simulink model "Sample594"  (R2021b)
settings: Solver=VariableStepAuto  StartTime=0.0  StopTime=10.0  RelTol=1e-3
undefined symbols (not defined in the file): DiscIntNeverNeededParam, magnitude, Newton, Raphson
libraries: simulink x402, pid_lib x98
(part 7 of 14)

== system Sample594/cfblk11/cfblk14/cfblk10/cfblk18 ==
  cfblk1 : Inport
  cfblk11 : Inport  Port=2
  cfblk12 : Inport  Port=3
  Action Port : ActionPort  ActionPortLabel=if(u1 >= 0)
  cfblk10 : Sin  TimeSource=Use external signal  SampleTime=0
  cfblk13 : Delay
  cfblk3 : DiscreteStateSpace  SampleTime=-1
  cfblk4 : pid_lib/PID Controller (2DOF)  Controller=PID  Form=Parallel  TimeDomain=Discrete-time  UseExternalTs=off  SampleTime=-1  IntegratorMethod=Forward Euler  FilterMethod=Forward Euler  ControllerParametersSource=internal  P=1  I=1  D=0  UseFilter=on  N=100  b=1  c=1  TunerSelectOption=Transfer Function Based (PID Tuner App)  InitialConditionSource=internal  InitialConditionForIntegrator=0  InitialConditionForFilter=0  DifferentiatorICPrevScaledInput=0  ExternalReset=none  TrackingMode=off  Kt=1  LimitOutput=off  SatLimitsSource=internal  UpperSaturationLimit=inf  LowerSaturationLimit=-inf  LinearizeAsGain=off  AntiWindupMode=none  Kb=1  POutMin=[]  POutMax=[]  IOutMin=[]  IOutMax=[]  DOutMin=[]  DOutMax=[]  NOutMin=[]  NOutMax=[]  bOutMin=[]  bOutMax=[]  cOutMin=[]  cOutMax=[]  SumOutMin=[]  SumOutMax=[]  SaturationOutMin=[]  SaturationOutMax=[]  PParamMin=[]  PParamMax=[]  IParamMin=[]  IParamMax=[]  DParamMin=[]  DParamMax=[]  NParamMin=[]  NParamMax=[]  bParamMin=[]  bParamMax=[]  cParamMin=[]  cParamMax=[]  KbParamMin=[]  KbParamMax=[]  KtParamMin=[]  KtParamMax=[]  KbOutMin=[]  KbOutMax=[]  KtOutMin=[]  KtOutMax=[]  IntegratorOutMin=[]  IntegratorOutMax=[]  FilterOutMin=[]  FilterOutMax=[]  SumI1OutMin=[]  SumI1OutMax=[]  SumI2OutMin=[]  SumI2OutMax=[]  SumI3OutMin=[]  SumI3OutMax=[]  SumI4OutMin=[]  SumI4OutMax=[]  SumDOutMin=[]  SumDOutMax=[]  Sum1OutMin=[]  Sum1OutMax=[]  Sum2OutMin=[]  Sum2OutMax=[]  Sum3OutMin=[]  Sum3OutMax=[]  DifferentiatorOutMin=[]  DifferentiatorOutMax=[]  FilterDiffOutCoefMin=[]  FilterDiffOutCoefMax=[]  ReciprocalOutMin=[]  ReciprocalOutMax=[]  SumDenOutMin=[]  SumDenOutMax=[]  SumNumOutMin=[]  SumNumOutMax=[]  DivideOutMin=[]  DivideOutMax=[]  UdiffTsProdOutMin=[]  UdiffTsProdOutMax=[]  NTsProdOutMin=[]  NTsProdOutMax=[]  UintegralTsProdOutMin=[]  UintegralTsProdOutMax=[]  UngainTsProdOutMin=[]  UngainTsProdOutMax=[]  IntegratorContinuousStateAttributes=''  IntegratorStateMustResolveToSignalObject=off  IntegratorRTWStateStorageClass=Auto  FilterContinuousStateAttributes=''  FilterStateMustResolveToSignalObject=off  FilterRTWStateStorageClass=Auto  ParallelPVariant=InternalParameters  IdealPVariant=Disabled  IVariant=InternalParameters  DVariant=InternalParameters  bVariant=InternalParameters  cVariant=InternalParameters  IntegratorVariant=Discrete  SatVariant=Disabled  AWVariant=Passthrough  PCopyVariant=Disabled  TRVariant=Disabled  FdbkBlocksVariant=Forward  IdealPFdbkVariant=Disabled  SatFdbkVariant=Disabled  DerivativeFilterVariant=ForwardEulerFilter  NVariant=InternalParameters  NCopyVariant=Disabled  FilterICVariant=InternalICsFilter  IntegratorICVariant=InternalICs  ExternalResetVariant=Disabled  TRSumVariant=Passthrough  SumFdbkVariant=Disabled  SumVariant=Sum_PID  TsampFilterVariant=InternalTs  TsampNgainVariant=Passthrough  TsampIntegralVariant=Passthrough  ExternalSaturationOutDataTypeStr=Inherit: Same as second input
      settings: SourceProductBaseCode=SL
  cfblk5 : simulink/Discrete/Transfer Fcn First Order  PoleZ=0.95  ICPrevOutput=0.0  DoSatur=off
  cfblk6 : Math  Operator=pow  SaturateOnIntegerOverflow=on
  cfblk7 : Gain  Gain=[178402085.468543]
  cfblk8 : Product
  cfblk9 : Trigonometry
  cfblk2 : Outport
  wires:
  cfblk1/1 -> cfblk10/1
  cfblk10/1 -> cfblk3/1, cfblk8/2
  cfblk3/1 -> cfblk2/1
  cfblk11/1 -> cfblk7/1
  cfblk9/1 -> cfblk4/1
  cfblk8/1 -> cfblk9/1
  cfblk12/1 -> cfblk6/1
  cfblk6/1 -> cfblk5/1
  cfblk7/1 -> cfblk6/2
  cfblk5/1 -> cfblk4/2
  cfblk4/1 -> cfblk13/1
  cfblk13/1 -> cfblk8/1

== system Sample594/cfblk11/cfblk14/cfblk10/cfblk19 ==
  cfblk1 : Inport
  cfblk7 : Inport  Port=2
  Action Port : ActionPort  ActionPortLabel=else
  cfblk3 : UnitDelay  SampleTime=-1  HasFrameUpgradeWarning=on
  cfblk4 : simulink/Discrete/Tapped Delay  vinit=0.0  samptime=-1  NumDelays=1  DelayOrder=Oldest  includeCurrent=off
  cfblk5 : PermuteDimensions
  cfblk6 : Polyval  Coefs=[ +2.081618890e-019, -1.441693666e-014, +4.719686976e-010, -8.536869453e-006, +1.621573104e-001, -8.087801117e+001 ]
  cfblk2 : Outport
  cfblk8 : Outport  Port=2
  wires:
  cfblk4/1 -> cfblk2/1
  cfblk1/1 -> cfblk3/1
  cfblk3/1 -> cfblk5/1
  cfblk7/1 -> cfblk6/1
  cfblk6/1 -> cfblk8/1
  cfblk5/1 -> cfblk4/1

== system Sample594/cfblk11/cfblk14/cfblk11/cfblk6 ==
  cfblk1 : Inport
  cfblk11 : Delay
  cfblk3 : simulink/Discrete/Tapped Delay  vinit=0.0  samptime=-1  NumDelays=1  DelayOrder=Oldest  includeCurrent=off
  cfblk4 : simulink/Discrete/Transfer Fcn Real Zero  ZeroZ=0.75  ICPrevInput=0.0  DoSatur=off
      settings: SourceProductBaseCode=SL
  cfblk5 : DiscreteTransferFcn
  cfblk6 : Math  Operator=magnitude^2  SaturateOnIntegerOverflow=on
  cfblk7 : UnaryMinus
  cfblk8 : DotProduct  InputSameDT=on  OutDataTypeStr=Inherit: Inherit via internal rule
  cfblk9 : ComplexToMagnitudeAngle
  cfblk2 : Outport
  cfblk10 : Outport  Port=2
  wires:
  cfblk1/1 -> cfblk4/1
  cfblk7/1 -> cfblk3/1
  cfblk9/1 -> cfblk8/1
  cfblk3/1 -> cfblk5/1
  cfblk4/1 -> cfblk9/1
  cfblk9/2 -> cfblk2/1
  cfblk6/1 -> cfblk7/1
  cfblk5/1 -> cfblk10/1, cfblk11/1
  cfblk8/1 -> cfblk6/1
  cfblk11/1 -> cfblk8/2

== system Sample594/cfblk11/cfblk14/cfblk11/cfblk7 ==
  cfblk1 : Inport
  cfblk9 : Inport  Port=2
  cfblk10 : Inport  Port=3
  cfblk11 : Inport  Port=4
  cfblk12 : Inport  Port=5
  cfblk3 : UnitDelay  SampleTime=-1  HasFrameUpgradeWarning=on
  cfblk4 : Rounding
  cfblk5 : Sqrt  Operator=rSqrt  AlgorithmType=Newton-Raphson  SaturateOnIntegerOverflow=on
  cfblk6 : Product  Inputs=**
  cfblk7 : Constant  Value=[-104542763.828041]  SampleTime=1
  cfblk8 : Constant  Value=[929127373.472288]  SampleTime=1
  cfblk2 : Outport
  cfblk13 : Outport  Port=2
  cfblk14 : Outport  Port=3
  wires:
  cfblk12/1 -> cfblk3/1
  cfblk8/1 -> cfblk13/1
  cfblk6/1 -> cfblk4/1
  cfblk10/1 -> cfblk6/1
  cfblk4/1 -> cfblk14/1
  cfblk9/1 -> cfblk2/1
  cfblk3/1 -> cfblk5/1
  cfblk7/1 -> cfblk6/2

== system Sample594/cfblk11/cfblk14/cfblk12/cfblk11 ==
  cfblk1 : Inport
  cfblk3 : UnitDelay  SampleTime=-1  HasFrameUpgradeWarning=on
  cfblk4 : DotProduct  InputSameDT=on  OutDataTypeStr=Inherit: Inherit via internal rule
  cfblk5 : Product  Inputs=**
  cfblk6 : simulink/Math Operations/MinMax Running Resettable  Function=min  vinit=0.0
  cfblk7 : Constant  Value=[-330095091.797810]  SampleTime=1
  cfblk2 : Outport
  wires:
  cfblk1/1 -> cfblk5/1, cfblk6/2
  cfblk6/1 -> cfblk3/1
  cfblk4/1 -> cfblk2/1
  cfblk7/1 -> cfblk5/2
  cfblk5/1 -> cfblk4/1, cfblk6/1
  cfblk3/1 -> cfblk4/2

== system Sample594/cfblk11/cfblk14/cfblk12/cfblk12 ==
  cfblk1 : Inport
  cfblk12 : Inport  Port=2
  cfblk10 : DotProduct  InputSameDT=on  OutDataTypeStr=Inherit: Inherit via internal rule
  cfblk11 : Constant  Value=[275284352.772494]  SampleTime=1
  cfblk17 : Delay
  cfblk18 : Delay
  cfblk3 : simulink/Discrete/Transfer Fcn Lead or Lag  PoleZ=0.95  ZeroZ=0.75  ICPrevOutput=0.0  ICPrevInput=0.0  DoSatur=off
      settings: SourceProductBaseCode=SL
  cfblk4 : simulink/Discrete/Tapped Delay  vinit=0.0  samptime=-1  NumDelays=1  DelayOrder=Oldest  includeCurrent=off
  cfblk5 : simulink/Discrete/Transfer Fcn Real Zero  ZeroZ=0.75  ICPrevInput=0.0  DoSatur=off
      settings: SourceProductBaseCode=SL
  cfblk6 : Assignment  DiagnosticForDimensions=Warning  IndexOptions=Index vector (dialog)  Indices=1  OutputSizes=1
  cfblk7 : MinMax  Function=max  Inputs=3
  cfblk8 : Sum  Inputs=+
  cfblk9 : Rounding
  cfblk2 : Outport
  cfblk13 : Outport  Port=2
  cfblk14 : Outport  Port=3
  cfblk15 : Outport  Port=4
  cfblk16 : Outport  Port=5
  wires:
  cfblk4/1 -> cfblk8/1
  cfblk1/1 -> cfblk9/1, cfblk6/2
  cfblk9/1 -> cfblk6/1, cfblk13/1
  cfblk7/1 -> cfblk4/1
  cfblk5/1 -> cfblk7/1
  cfblk10/1 -> cfblk16/1, cfblk7/3
  cfblk12/1 -> cfblk5/1, cfblk3/1
  cfblk11/1 -> cfblk14/1
  cfblk3/1 -> cfblk10/1
  cfblk8/1 -> cfblk2/1, cfblk17/1, cfblk18/1
  cfblk6/1 -> cfblk15/1
  cfblk17/1 -> cfblk10/2
  cfblk18/1 -> cfblk7/2

== system Sample594/cfblk11/cfblk14/cfblk12/cfblk13 ==
  cfblk1 : Inport
  cfblk9 : Inport  Port=2
  cfblk3 : simulink/Discrete/Transfer Fcn Lead or Lag  PoleZ=0.95  ZeroZ=0.75  ICPrevOutput=0.0  ICPrevInput=0.0  DoSatur=off
      settings: SourceProductBaseCode=SL
  cfblk4 : DiscreteStateSpace  SampleTime=-1
  cfblk5 : DiscreteIntegrator  SampleTime=-1  ICPrevOutput=DiscIntNeverNeededParam  ICPrevScaledInput=DiscIntNeverNeededParam
  cfblk6 : Gain  Gain=[347826700.249157]
  cfblk7 : Sqrt  Operator=rSqrt  AlgorithmType=Newton-Raphson  SaturateOnIntegerOverflow=on
  cfblk8 : Constant  Value=[-978671708.765340]  SampleTime=1
  cfblk2 : Outport
  wires:
  cfblk5/1 -> cfblk6/1
  cfblk1/1 -> cfblk4/1
  cfblk8/1 -> cfblk7/1
  cfblk3/1 -> cfblk2/1
  cfblk9/1 -> cfblk3/1
  cfblk4/1 -> cfblk5/1

== system Sample594/cfblk11/cfblk14/cfblk12/cfblk18 ==
  cfblk1 : Inport
  cfblk10 : Inport  Port=2
  Action Port : ActionPort  ActionPortLabel=if(u1 >= 0)
  cfblk3 : Trigonometry
  cfblk4 : Math  Operator=conj  SaturateOnIntegerOverflow=on
  cfblk5 : Polyval  Coefs=[ +2.081618890e-019, -1.441693666e-014, +4.719686976e-010, -8.536869453e-006, +1.621573104e-001, -8.087801117e+001 ]
  cfblk6 : Gain  Gain=[899770617.294449]
  cfblk7 : Rounding
  cfblk8 : ComplexToRealImag
  cfblk9 : Constant  Value=[-198075517.030660]  SampleTime=1
  cfblk2 : Outport
  wires:
  cfblk10/1 -> cfblk4/1
  cfblk7/1 -> cfblk8/1
  cfblk8/1 -> cfblk6/1
  cfblk9/1 -> cfblk3/1
  cfblk5/1 -> cfblk7/1
  cfblk3/1 -> cfblk5/1
  cfblk4/1 -> cfblk2/1

== system Sample594/cfblk11/cfblk14/cfblk12/cfblk19 ==
  cfblk1 : Inport
  cfblk17 : Inport  Port=2
  Action Port : ActionPort  ActionPortLabel=else
  cfblk10 : Sum  Inputs=|++
  cfblk11 : DotProduct  InputSameDT=on  OutDataTypeStr=Inherit: Inherit via internal rule
  cfblk12 : Polyval  Coefs=[ +2.081618890e-019, -1.441693666e-014, +4.719686976e-010, -8.536869453e-006, +1.621573104e-001, -8.087801117e+001 ]
  cfblk13 : UnaryMinus
  cfblk14 : Math  Operator=hermitian  SaturateOnIntegerOverflow=on
  cfblk15 : Constant  Value=[774872424.873836]  SampleTime=1
  cfblk16 : Constant  Value=[-500925390.501098]  SampleTime=1
  cfblk18 : Delay
  cfblk19 : Delay
  cfblk3 : DiscreteTransferFcn
  cfblk4 : Delay
  cfblk5 : simulink/Discrete/Transfer Fcn First Order  PoleZ=0.95  ICPrevOutput=0.0  DoSatur=off
  cfblk6 : simulink/Discrete/Difference  ICPrevInput=0.0  OutMin=[]  OutMax=[]  OutDataTypeStr=Inherit: Inherit via back propagation  OutDataType=fixdt(1, 16)  OutScaling=2^-10  DoSatur=off
  cfblk7 : DiscreteIntegrator  SampleTime=-1  ICPrevOutput=DiscIntNeverNeededParam  ICPrevScaledInput=DiscIntNeverNeededParam
  cfblk8 : Math  Operator=10^u  SaturateOnIntegerOverflow=on
  cfblk9 : Math  Operator=log  SaturateOnIntegerOverflow=on
  cfblk2 : Outport
  wires:
  cfblk14/1 -> cfblk12/1
  cfblk13/1 -> cfblk6/1
  cfblk5/1 -> cfblk13/1
  cfblk4/1 -> cfblk7/1
  cfblk15/1 -> cfblk5/1
  cfblk3/1 -> cfblk9/1
  cfblk10/1 -> cfblk14/1
  cfblk1/1 -> cfblk3/1
  cfblk9/1 -> cfblk2/1
  cfblk16/1 -> cfblk10/2
  cfblk6/1 -> cfblk4/1
  cfblk17/1 -> cfblk11/1
  cfblk8/1 -> cfblk11/2
  cfblk11/1 -> cfblk18/1
  cfblk18/1 -> cfblk8/1
  cfblk12/1 -> cfblk19/1
  cfblk19/1 -> cfblk10/1

== system Sample594/cfblk11/cfblk15/cfblk7/cfblk7 ==
  cfblk1 : Inport
  cfblk9 : Inport  Port=2
  cfblk10 : Inport  Port=3
  cfblk12 : Delay
  cfblk3 : Delay  DelayLengthSource=Input port
      settings: InputPortMap=u0,p1
  cfblk4 : DiscreteIntegrator  SampleTime=-1  ICPrevOutput=DiscIntNeverNeededParam  ICPrevScaledInput=DiscIntNeverNeededParam
  cfblk5 : Rounding
  cfblk6 : simulink/Math Operations/Slider Gain  gain=1  low=0  high=2
  cfblk7 : Polyval  Coefs=[ +2.081618890e-019, -1.441693666e-014, +4.719686976e-010, -8.536869453e-006, +1.621573104e-001, -8.087801117e+001 ]
  cfblk8 : Constant  Value=[162624485.330461]  SampleTime=1
  cfblk2 : Outport
  cfblk11 : Outport  Port=2
  wires:
  cfblk5/1 -> cfblk7/1
  cfblk9/1 -> cfblk3/1
  cfblk6/1 -> cfblk5/1
  cfblk8/1 -> cfblk4/1
  cfblk3/1 -> cfblk6/1
  cfblk4/1 -> cfblk11/1
  cfblk1/1 -> cfblk2/1
  cfblk7/1 -> cfblk12/1
  cfblk12/1 -> cfblk3/2

== system Sample594/cfblk11/cfblk15/cfblk8/cfblk13 ==
  cfblk1 : Inport
  cfblk9 : Inport  Port=2
  Action Port : ActionPort  ActionPortLabel=if(u1 >= 0)
  cfblk3 : Rounding
  cfblk4 : Product  Inputs=*
  cfblk5 : Trigonometry
  cfblk6 : MinMax  Function=max  Inputs=2
  cfblk7 : Trigonometry
  cfblk8 : Constant  Value=[-890306196.442185]  SampleTime=1
  cfblk2 : Outport
  cfblk10 : Outport  Port=2
  wires:
  cfblk4/1 -> cfblk5/1
  cfblk7/1 -> cfblk6/1
  cfblk9/1 -> cfblk7/1
  cfblk5/1 -> cfblk3/1
  cfblk8/1 -> cfblk10/1
  cfblk3/1 -> cfblk2/1
  cfblk6/1 -> cfblk4/1
  cfblk1/1 -> cfblk6/2

== system Sample594/cfblk11/cfblk15/cfblk8/cfblk14 ==
  cfblk1 : Inport
  cfblk13 : Inport  Port=2
  cfblk14 : Inport  Port=3
  cfblk15 : Inport  Port=4
  Action Port : ActionPort  ActionPortLabel=else
  cfblk10 : ComplexToMagnitudeAngle
  cfblk11 : Abs
  cfblk12 : Constant  Value=[662032914.348049]  SampleTime=1
  cfblk3 : simulink/Discrete/Transfer Fcn Real Zero  ZeroZ=0.75  ICPrevInput=0.0  DoSatur=off
      settings: SourceProductBaseCode=SL
  cfblk4 : UnitDelay  SampleTime=-1  HasFrameUpgradeWarning=on
  cfblk5 : simulink/Discrete/Transfer Fcn Lead or Lag  PoleZ=0.95  ZeroZ=0.75  ICPrevOutput=0.0  ICPrevInput=0.0  DoSatur=off
      settings: SourceProductBaseCode=SL
  cfblk6 : Product  Inputs=*
  cfblk7 : Sum  Inputs=+
  cfblk8 : Squeeze
  cfblk9 : Trigonometry
  cfblk2 : Outport
  cfblk16 : Outport  Port=2
  wires:
  cfblk1/1 -> cfblk9/1
  cfblk4/1 -> cfblk11/1
  cfblk9/1 -> cfblk5/1
  cfblk15/1 -> cfblk4/1
  cfblk7/1 -> cfblk10/1
  cfblk10/1 -> cfblk8/1
  cfblk12/1 -> cfblk3/1
  cfblk13/1 -> cfblk16/1
  cfblk5/1 -> cfblk7/1
  cfblk14/1 -> cfblk6/1
  cfblk3/1 -> cfblk2/1

== system Sample594/cfblk11/cfblk15/cfblk8/cfblk7 ==
  cfblk1 : Inport
  cfblk8 : Inport  Port=2
  cfblk9 : Inport  Port=3
  cfblk10 : Inport  Port=4
  cfblk11 : Inport  Port=5
  cfblk12 : Inport  Port=6
  cfblk3 : Gain  Gain=[19992525.824137]
  cfblk4 : Product  Inputs=**
  cfblk5 : simulink/Math Operations/Slider Gain  gain=1  low=0  high=2
  cfblk6 : Rounding
  cfblk7 : MinMax  Function=max  Inputs=3
  cfblk2 : Outport
  wires:
  cfblk4/1 -> cfblk2/1
  cfblk9/1 -> cfblk6/1
  cfblk12/1 -> cfblk5/1
  cfblk3/1 -> cfblk7/1
  cfblk5/1 -> cfblk7/2
  cfblk7/1 -> cfblk4/1
  cfblk1/1 -> cfblk7/3
  cfblk11/1 -> cfblk4/2
  cfblk8/1 -> cfblk3/1

== system Sample594/cfblk11/cfblk15/cfblk8/cfblk8 ==
  cfblk1 : Inport
  cfblk7 : Inport  Port=2
  cfblk8 : Inport  Port=3
  cfblk3 : simulink/Discrete/Tapped Delay  vinit=0.0  samptime=-1  NumDelays=1  DelayOrder=Oldest  includeCurrent=off
  cfblk4 : PermuteDimensions
  cfblk5 : Constant  Value=[843769365.863623]  SampleTime=1
  cfblk6 : Constant  Value=[155937081.446852]  SampleTime=1
  cfblk2 : Outport
  cfblk9 : Outport  Port=2
  wires:
  cfblk7/1 -> cfblk3/1
  cfblk6/1 -> cfblk2/1
  cfblk1/1 -> cfblk4/1
  cfblk8/1 -> cfblk9/1

== system Sample594/cfblk11/cfblk15/cfblk8/cfblk9 ==
  cfblk1 : Inport
  cfblk10 : Delay
  cfblk3 : Delay  DelayLengthSource=Input port
      settings: InputPortMap=u0,p1
  cfblk4 : Sin  TimeSource=Use external signal  SampleTime=0
  cfblk5 : simulink/Math Operations/Slider Gain  gain=1  low=0  high=2
  cfblk6 : Bias  Bias=[350296678.166723]
  cfblk7 : DotProduct  InputSameDT=on  OutDataTypeStr=Inherit: Inherit via internal rule
  cfblk8 : Product  Inputs=*
  cfblk2 : Outport
  cfblk9 : Outport  Port=2
  wires:
  cfblk7/1 -> cfblk2/1
  cfblk8/1 -> cfblk9/1
  cfblk3/1 -> cfblk6/1, cfblk8/1
  cfblk1/1 -> cfblk3/1, cfblk7/2, cfblk5/1
  cfblk6/1 -> cfblk4/1
  cfblk5/1 -> cfblk7/1
  cfblk4/1 -> cfblk10/1
  cfblk10/1 -> cfblk3/2

== system Sample594/cfblk11/cfblk18/cfblk10/cfblk10 ==
  cfblk1 : Inport
  cfblk11 : Inport  Port=2
  cfblk12 : Inport  Port=3
  cfblk10 : Constant  Value=[-338781985.108601]  SampleTime=1
  cfblk13 : Delay
  cfblk3 : DiscreteStateSpace  SampleTime=-1
  cfblk4 : simulink/Discrete/Transfer Fcn First Order  PoleZ=0.95  ICPrevOutput=0.0  DoSatur=off
  cfblk5 : Delay  DelayLengthSource=Input port
      settings: InputPortMap=u0,p1
  cfblk6 : DotProduct  InputSameDT=on  OutDataTypeStr=Inherit: Inherit via internal rule
  cfblk7 : Signum
  cfblk8 : Product  Inputs=*
  cfblk9 : Constant  Value=[-590553005.063155]  SampleTime=1
  cfblk2 : Outport
  wires:
  cfblk3/1 -> cfblk8/1
  cfblk8/1 -> cfblk5/1
  cfblk11/1 -> cfblk2/1
  cfblk6/1 -> cfblk7/1
  cfblk5/1 -> cfblk6/2
  cfblk10/1 -> cfblk4/1
  cfblk9/1 -> cfblk3/1
  cfblk12/1 -> cfblk5/2
  cfblk7/1 -> cfblk13/1
  cfblk13/1 -> cfblk6/1

== system Sample594/cfblk11/cfblk18/cfblk10/cfblk11 ==
  cfblk1 : Inport
  cfblk8 : Inport  Port=2
  cfblk9 : Inport  Port=3
  cfblk10 : Inport  Port=4
  cfblk11 : Inport  Port=5
  cfblk3 : simulink/Discrete/Transfer Fcn Lead or Lag  PoleZ=0.95  ZeroZ=0.75  ICPrevOutput=0.0  ICPrevInput=0.0  DoSatur=off
      settings: SourceProductBaseCode=SL
  cfblk4 : Product
  cfblk5 : Bias  Bias=[134923458.649195]
  cfblk6 : PermuteDimensions
  cfblk7 : MinMax  Function=max  Inputs=2
  cfblk2 : Outport
  cfblk12 : Outport  Port=2
  wires:
  cfblk1/1 -> cfblk7/1
  cfblk5/1 -> cfblk3/1
  cfblk3/1 -> cfblk12/1
  cfblk7/1 -> cfblk2/1
  cfblk4/1 -> cfblk7/2
  cfblk8/1 -> cfblk6/1
  cfblk10/1 -> cfblk5/1
  cfblk9/1 -> cfblk4/1
  cfblk6/1 -> cfblk4/2

== system Sample594/cfblk11/cfblk18/cfblk10/cfblk12 ==
  cfblk1 : Inport
  cfblk12 : Inport  Port=2
  cfblk13 : Inport  Port=3
  cfblk14 : Inport  Port=4
  cfblk10 : simulink/Math Operations/MinMax Running Resettable  Function=min  vinit=0.0
  cfblk11 : Constant  Value=[904304465.942698]  SampleTime=1
  cfblk3 : simulink/Discrete/Difference  ICPrevInput=0.0  OutMin=[]  OutMax=[]  OutDataTypeStr=Inherit: Inherit via back propagation  OutDataType=fixdt(1, 16)  OutScaling=2^-10  DoSatur=off
  cfblk4 : DiscreteIntegrator  SampleTime=-1  ICPrevOutput=DiscIntNeverNeededParam  ICPrevScaledInput=DiscIntNeverNeededParam
  cfblk5 : DiscreteFilter
  cfblk6 : Product  Inputs=**
  cfblk7 : Assignment  DiagnosticForDimensions=Warning  IndexOptions=Index vector (dialog)  Indices=1  OutputSizes=1
  cfblk8 : Product  Inputs=*
  cfblk9 : ComplexToMagnitudeAngle
  cfblk2 : Outport
  cfblk15 : Outport  Port=2
  cfblk16 : Outport  Port=3
  wires:
  cfblk14/1 -> cfblk6/1
  cfblk6/1 -> cfblk5/1
  cfblk1/1 -> cfblk8/1
  cfblk5/1 -> cfblk9/1
  cfblk9/1 -> cfblk7/1
  cfblk7/1 -> cfblk10/1
  cfblk9/2 -> cfblk15/1
  cfblk11/1 -> cfblk4/1
  cfblk13/1 -> cfblk6/2
  cfblk12/1 -> cfblk7/2
  cfblk3/1 -> cfblk16/1
  cfblk4/1 -> cfblk10/2
  cfblk10/1 -> cfblk2/1
  cfblk8/1 -> cfblk3/1

== system Sample594/cfblk11/cfblk18/cfblk10/cfblk8 ==
  cfblk1 : Inport
  cfblk8 : Inport  Port=2
  cfblk9 : Inport  Port=3
  cfblk10 : Inport  Port=4
  cfblk3 : DiscreteTransferFcn
  cfblk4 : Sum  Inputs=+-
  cfblk5 : Gain  Gain=[349576824.036338]
  cfblk6 : Constant  Value=[-943928355.856876]  SampleTime=1
  cfblk7 : Constant  Value=[-837650532.440236]  SampleTime=1
  cfblk2 : Outport
  wires:
  cfblk6/1 -> cfblk5/1
  cfblk7/1 -> cfblk3/1
  cfblk1/1 -> cfblk4/1
  cfblk8/1 -> cfblk2/1
  cfblk3/1 -> cfblk4/2

== system Sample594/cfblk11/cfblk18/cfblk10/cfblk9 ==
  cfblk1 : Inport
  cfblk12 : Inport  Port=2
  cfblk13 : Inport  Port=3
  cfblk14 : Inport  Port=4
  cfblk10 : Sum  Inputs=|++
  cfblk11 : ComplexToMagnitudeAngle
  cfblk16 : Delay
  cfblk3 : Delay
  cfblk4 : DiscreteFir
  cfblk5 : simulink/Discrete/Transfer Fcn First Order  PoleZ=0.95  ICPrevOutput=0.0  DoSatur=off
  cfblk6 : Assignment  DiagnosticForDimensions=Warning  IndexOptions=Index vector (dialog)  Indices=1  OutputSizes=1
  cfblk7 : Squeeze
  cfblk8 : ComplexToMagnitudeAngle
  cfblk9 : Signum
  cfblk2 : Outport
  cfblk15 : Outport  Port=2
  wires:
  cfblk5/1 -> cfblk10/1
  cfblk12/1 -> cfblk3/1
  cfblk1/1 -> cfblk7/1
  cfblk13/1 -> cfblk9/1
  cfblk7/1 -> cfblk6/1
  cfblk9/1 -> cfblk2/1
  cfblk6/1 -> cfblk10/2
  cfblk3/1 -> cfblk4/1
  cfblk14/1 -> cfblk6/2
  cfblk11/2 -> cfblk5/1
  cfblk8/1 -> cfblk15/1
  cfblk8/2 -> cfblk11/1
  cfblk11/1 -> cfblk16/1
  cfblk16/1 -> cfblk8/1

== system Sample594/cfblk11/cfblk18/cfblk11/cfblk10 ==
  cfblk1 : Inport
  cfblk10 : Inport  Port=2
  cfblk11 : Delay
  cfblk3 : DiscreteZeroPole  Poles=[0 0.5]  Gain=1  SampleTime=-1
  cfblk4 : Delay  DelayLengthSource=Input port
      settings: InputPortMap=u0,p1
  cfblk5 : simulink/Discrete/Transfer Fcn First Order  PoleZ=0.95  ICPrevOutput=0.0  DoSatur=off
  cfblk6 : Abs
  cfblk7 : Product  Inputs=**
  cfblk8 : Constant  Value=[-310177978.418347]  SampleTime=1
  cfblk9 : Constant  Value=[601529275.309641]  SampleTime=1
  cfblk2 : Outport
  wires:
  cfblk8/1 -> cfblk7/1
  cfblk10/1 -> cfblk4/1
  cfblk9/1 -> cfblk3/1
  cfblk1/1 -> cfblk2/1
  cfblk4/1 -> cfblk6/1
  cfblk6/1 -> cfblk5/1
  cfblk3/1 -> cfblk7/2
  cfblk5/1 -> cfblk11/1
  cfblk11/1 -> cfblk4/2

== system Sample594/cfblk11/cfblk18/cfblk11/cfblk11 ==
  cfblk1 : Inport
  cfblk16 : Inport  Port=2
  cfblk10 : Product  Inputs=**
  cfblk11 : Product  Inputs=**
  cfblk12 : PermuteDimensions
  cfblk13 : Constant  Value=[169176575.139940]  SampleTime=1
  cfblk14 : Constant  Value=[927732317.586605]  SampleTime=1
  cfblk15 : Constant  Value=[843097676.908969]  SampleTime=1
  cfblk18 : Delay
  cfblk3 : Delay
  cfblk4 : simulink/Discrete/Tapped Delay  vinit=0.0  samptime=-1  NumDelays=1  DelayOrder=Oldest  includeCurrent=off
  cfblk5 : simulink/Discrete/Transfer Fcn First Order  PoleZ=0.95  ICPrevOutput=0.0  DoSatur=off
  cfblk6 : DiscreteTransferFcn
  cfblk7 : DiscreteTransferFcn
  cfblk8 : Rounding
  cfblk9 : Reshape
  cfblk2 : Outport
  cfblk17 : Outport  Port=2
  wires:
  cfblk3/1 -> cfblk17/1
  cfblk11/1 -> cfblk4/1
  cfblk16/1 -> cfblk7/1
  cfblk15/1 -> cfblk9/1
  cfblk5/1 -> cfblk6/1
  cfblk7/1 -> cfblk3/1
  cfblk4/1 -> cfblk12/1
  cfblk8/1 -> cfblk10/1
  cfblk9/1 -> cfblk10/2
  cfblk12/1 -> cfblk5/1
  cfblk6/1 -> cfblk2/1
  cfblk13/1 -> cfblk11/1
  cfblk1/1 -> cfblk11/2
  cfblk10/1 -> cfblk18/1
  cfblk18/1 -> cfblk8/1

== system Sample594/cfblk11/cfblk18/cfblk11/cfblk8 ==
  cfblk1 : Inport
  cfblk6 : Inport  Port=2
  cfblk7 : Inport  Port=3
  cfblk3 : DiscreteTransferFcn
  cfblk4 : Math  Operator=hypot  SaturateOnIntegerOverflow=on
  cfblk5 : DotProduct  InputSameDT=on  OutDataTypeStr=Inherit: Inherit via internal rule
  cfblk8 : Delay
  cfblk2 : Outport
  wires:
  cfblk3/1 -> cfblk4/1
  cfblk6/1 -> cfblk4/2
  cfblk1/1 -> cfblk2/1
  cfblk4/1 -> cfblk5/1
  cfblk7/1 -> cfblk5/2
  cfblk5/1 -> cfblk8/1
  cfblk8/1 -> cfblk3/1

== system Sample594/cfblk11/cfblk18/cfblk11/cfblk9 ==
  cfblk1 : Inport
  cfblk9 : Inport  Port=2
  cfblk10 : Inport  Port=3
  cfblk11 : Inport  Port=4
  cfblk12 : Inport  Port=5
  cfblk3 : simulink/Discrete/Transfer Fcn First Order  PoleZ=0.95  ICPrevOutput=0.0  DoSatur=off
  cfblk4 : Trigonometry
  cfblk5 : UnaryMinus
  cfblk6 : Sqrt  SaturateOnIntegerOverflow=on
  cfblk7 : Sum  Inputs=--
  cfblk8 : Constant  Value=[733536568.390652]  SampleTime=1
  cfblk2 : Outport
  wires:
  cfblk3/1 -> cfblk6/1
  cfblk4/1 -> cfblk5/1
  cfblk11/1 -> cfblk4/1
  cfblk10/1 -> cfblk2/1
  cfblk5/1 -> cfblk7/1
  cfblk7/1 -> cfblk3/1
  cfblk9/1 -> cfblk7/2

== system Sample594/cfblk11/cfblk18/cfblk9/cfblk10 ==
  cfblk1 : Inport
  cfblk9 : Inport  Port=2
  cfblk3 : Delay  ShowEnablePort=on
      settings: InputPortMap=u0,e6
  cfblk4 : Delay  DelayLengthSource=Input port
      settings: InputPortMap=u0,p1
  cfblk5 : UnaryMinus
  cfblk6 : simulink/Math Operations/MinMax Running Resettable  Function=min  vinit=0.0
  cfblk7 : Abs
  cfblk8 : Reshape
  cfblk2 : Outport
  cfblk10 : Outport  Port=2
  cfblk11 : Outport  Port=3
  wires:
  cfblk8/1 -> cfblk4/1, cfblk5/1, cfblk3/2
  cfblk7/1 -> cfblk6/1
  cfblk9/1 -> cfblk8/1
  cfblk5/1 -> cfblk6/2
  cfblk1/1 -> cfblk4/2
  cfblk4/1 -> cfblk7/1, cfblk2/1
  cfblk6/1 -> cfblk3/1, cfblk10/1
  cfblk3/1 -> cfblk11/1

== system Sample594/cfblk11/cfblk18/cfblk9/cfblk11 ==
  cfblk1 : Inport
  cfblk3 : DiscreteFir
  cfblk4 : simulink/Discrete/Transfer Fcn Lead or Lag  PoleZ=0.95  ZeroZ=0.75  ICPrevOutput=0.0  ICPrevInput=0.0  DoSatur=off
      settings: SourceProductBaseCode=SL
  cfblk5 : simulink/Discrete/Tapped Delay  vinit=0.0  samptime=-1  NumDelays=1  DelayOrder=Oldest  includeCurrent=off
  cfblk6 : Signum
  cfblk7 : Gain  Gain=[390625445.766554]
  cfblk8 : Constant  Value=[-352259615.704851]  SampleTime=1
  cfblk9 : Constant  Value=[558965235.639887]  SampleTime=1
  cfblk2 : Outport
  wires:
  cfblk3/1 -> cfblk5/1
  cfblk6/1 -> cfblk2/1
  cfblk1/1 -> cfblk7/1
  cfblk4/1 -> cfblk3/1
  cfblk7/1 -> cfblk6/1
  cfblk9/1 -> cfblk4/1

== system Sample594/cfblk11/cfblk19/cfblk6/cfblk10 ==
  cfblk1 : Inport
  cfblk15 : Inport  Port=2
  cfblk16 : Inport  Port=3
  cfblk10 : PermuteDimensions
  cfblk11 : Rounding
  cfblk12 : Gain  Gain=[-291401441.009689]
  cfblk13 : Product  Inputs=**
  cfblk14 : Constant  Value=[265543528.572169]  SampleTime=1
  cfblk18 : Delay
  cfblk19 : Delay
  cfblk3 : DiscreteIntegrator  SampleTime=-1  ICPrevOutput=DiscIntNeverNeededParam  ICPrevScaledInput=DiscIntNeverNeededParam
  cfblk4 : DiscreteFir
  cfblk5 : DiscreteTransferFcn
  cfblk6 : Delay  ShowEnablePort=on
      settings: InputPortMap=u0,e6
  cfblk7 : Product  Inputs=**
  cfblk8 : Assignment  DiagnosticForDimensions=Warning  IndexOptions=Index vector (dialog)  Indices=1  OutputSizes=1
  cfblk9 : UnaryMinus
  cfblk2 : Outport
  cfblk17 : Outport  Port=2
  wires:
  cfblk1/1 -> cfblk5/1
  cfblk6/1 -> cfblk11/1
  cfblk16/1 -> cfblk8/2
  cfblk14/1 -> cfblk12/1
  cfblk9/1 -> cfblk17/1
  cfblk13/1 -> cfblk4/1, cfblk18/1
  cfblk5/1 -> cfblk3/1, cfblk9/1
  cfblk4/1 -> cfblk2/1
  cfblk11/1 -> cfblk7/1
  cfblk8/1 -> cfblk10/1
  cfblk3/1 -> cfblk6/1
  cfblk7/1 -> cfblk13/1
  cfblk12/1 -> cfblk13/2
  cfblk15/1 -> cfblk7/2
  cfblk18/1 -> cfblk6/2
  cfblk10/1 -> cfblk19/1
  cfblk19/1 -> cfblk8/1

== system Sample594/cfblk11/cfblk19/cfblk6/cfblk8 ==
  cfblk1 : Inport
  cfblk8 : Inport  Port=2
  cfblk9 : Inport  Port=3
  cfblk3 : Delay  ShowEnablePort=on
      settings: InputPortMap=u0,e6
  cfblk4 : Delay  ShowEnablePort=on
      settings: InputPortMap=u0,e6
  cfblk5 : PermuteDimensions
  cfblk6 : Sqrt  SaturateOnIntegerOverflow=on
  cfblk7 : Constant  Value=[875759112.050450]  SampleTime=1
  cfblk2 : Outport
  cfblk10 : Outport  Port=2
  cfblk11 : Outport  Port=3
  wires:
  cfblk4/1 -> cfblk6/1
  cfblk9/1 -> cfblk2/1
  cfblk7/1 -> cfblk3/1
  cfblk1/1 -> cfblk4/1
  cfblk6/1 -> cfblk3/2
  cfblk3/1 -> cfblk10/1
  cfblk8/1 -> cfblk5/1
  cfblk5/1 -> cfblk11/1, cfblk4/2

== system Sample594/cfblk11/cfblk19/cfblk6/cfblk9 ==
  cfblk1 : Inport
  cfblk10 : Inport  Port=2
  cfblk3 : UnitDelay  SampleTime=-1  HasFrameUpgradeWarning=on
  cfblk4 : simulink/Discrete/Difference  ICPrevInput=0.0  OutMin=[]  OutMax=[]  OutDataTypeStr=Inherit: Inherit via back propagation  OutDataType=fixdt(1, 16)  OutScaling=2^-10  DoSatur=off
  cfblk5 : DiscreteFir
  cfblk6 : Squeeze
  cfblk7 : Squeeze
  cfblk8 : Sum  Inputs=+
  cfblk9 : Constant  Value=[418992866.198597]  SampleTime=1
  cfblk2 : Outport
  wires:
  cfblk10/1 -> cfblk3/1
  cfblk6/1 -> cfblk8/1
  cfblk3/1 -> cfblk6/1
  cfblk7/1 -> cfblk5/1
  cfblk1/1 -> cfblk2/1
  cfblk8/1 -> cfblk7/1
  cfblk5/1 -> cfblk4/1

== system Sample594/cfblk11/cfblk19/cfblk7/cfblk5 ==
  cfblk1 : Inport
  cfblk7 : Inport  Port=2
  cfblk3 : simulink/Discrete/Tapped Delay  vinit=0.0  samptime=-1  NumDelays=1  DelayOrder=Oldest  includeCurrent=off
  cfblk4 : DiscreteStateSpace  SampleTime=-1
  cfblk5 : Math  Operator=square  SaturateOnIntegerOverflow=on
  cfblk6 : Constant  Value=[772451761.004515]  SampleTime=1
  cfblk2 : Outport
  cfblk8 : Outport  Port=2
  wires:
  cfblk6/1 -> cfblk8/1
  cfblk1/1 -> cfblk4/1
  cfblk7/1 -> cfblk3/1
  cfblk4/1 -> cfblk5/1
  cfblk5/1 -> cfblk2/1

== system Sample594/cfblk11/cfblk19/cfblk7/cfblk6 ==
  cfblk1 : Inport
  cfblk10 : Constant  Value=[901565639.160194]  SampleTime=1
  cfblk11 : Delay
  cfblk3 : pid_lib/PID Controller  Controller=PID  Form=Parallel  TimeDomain=Discrete-time  UseExternalTs=off  SampleTime=-1  IntegratorMethod=Forward Euler  FilterMethod=Forward Euler  ControllerParametersSource=internal  P=1  I=1  D=0  UseFilter=on  N=100  TunerSelectOption=Transfer Function Based (PID Tuner App)  InitialConditionSource=internal  InitialConditionForIntegrator=0  InitialConditionForFilter=0  DifferentiatorICPrevScaledInput=0  ExternalReset=none  TrackingMode=off  Kt=1  LimitOutput=off  SatLimitsSource=internal  UpperSaturationLimit=inf  LowerSaturationLimit=-inf  LinearizeAsGain=off  AntiWindupMode=none  Kb=1  POutMin=[]  POutMax=[]  IOutMin=[]  IOutMax=[]  DOutMin=[]  DOutMax=[]  NOutMin=[]  NOutMax=[]  SumOutMin=[]  SumOutMax=[]  SaturationOutMin=[]  SaturationOutMax=[]  PParamMin=[]  PParamMax=[]  IParamMin=[]  IParamMax=[]  DParamMin=[]  DParamMax=[]  NParamMin=[]  NParamMax=[]  KbParamMin=[]  KbParamMax=[]  KtParamMin=[]  KtParamMax=[]  KbOutMin=[]  KbOutMax=[]  KtOutMin=[]  KtOutMax=[]  IntegratorOutMin=[]  IntegratorOutMax=[]  FilterOutMin=[]  FilterOutMax=[]  SumI1OutMin=[]  SumI1OutMax=[]  SumI2OutMin=[]  SumI2OutMax=[]  SumI3OutMin=[]  SumI3OutMax=[]  SumI4OutMin=[]  SumI4OutMax=[]  SumDOutMin=[]  SumDOutMax=[]  DifferentiatorOutMin=[]  DifferentiatorOutMax=[]  FilterDiffOutCoefMin=[]  FilterDiffOutCoefMax=[]  ReciprocalOutMin=[]  ReciprocalOutMax=[]  SumDenOutMin=[]  SumDenOutMax=[]  SumNumOutMin=[]  SumNumOutMax=[]  DivideOutMin=[]  DivideOutMax=[]  UdiffTsProdOutMin=[]  UdiffTsProdOutMax=[]  NTsProdOutMin=[]  NTsProdOutMax=[]  UintegralTsProdOutMin=[]  UintegralTsProdOutMax=[]  UngainTsProdOutMin=[]  UngainTsProdOutMax=[]  IntegratorContinuousStateAttributes=''  IntegratorStateMustResolveToSignalObject=off  IntegratorRTWStateStorageClass=Auto  FilterContinuousStateAttributes=''  FilterStateMustResolveToSignalObject=off  FilterRTWStateStorageClass=Auto  ParallelPVariant=InternalParameters  IdealPVariant=Disabled  IVariant=InternalParameters  DVariant=InternalParameters  IntegratorVariant=Discrete  SatVariant=Disabled  AWVariant=Passthrough  PCopyVariant=Disabled  TRVariant=Disabled  FdbkBlocksVariant=Forward  IdealPFdbkVariant=Disabled  SatFdbkVariant=Disabled  DerivativeFilterVariant=ForwardEulerFilter  NVariant=InternalParameters  NCopyVariant=Disabled  FilterICVariant=InternalICsFilter  IntegratorICVariant=InternalICs  ExternalResetVariant=Disabled  TRSumVariant=Passthrough  SumFdbkVariant=Disabled  SumVariant=Sum_PID  TsampFilterVariant=InternalTs  TsampNgainVariant=Passthrough  TsampIntegralVariant=Passthrough  ExternalSaturationOutDataTypeStr=Inherit: Same as second input
  cfblk4 : DiscreteTransferFcn
  cfblk5 : Sum  Inputs=+
  cfblk6 : ComplexToRealImag
  cfblk7 : Sin  TimeSource=Use external signal  SampleTime=0
  cfblk8 : Sin  TimeSource=Use external signal  SampleTime=0
  cfblk9 : MinMax
  cfblk2 : Outport
  wires:
  cfblk10/1 -> cfblk3/1
  cfblk3/1 -> cfblk5/1
  cfblk6/1 -> cfblk8/1
  cfblk9/1 -> cfblk2/1
  cfblk6/2 -> cfblk7/1
  cfblk7/1 -> cfblk4/1
  cfblk5/1 -> cfblk9/1
  cfblk8/1 -> cfblk11/1
  cfblk11/1 -> cfblk6/1

== system Sample594/cfblk11/cfblk19/cfblk7/cfblk7 ==
  cfblk1 : Inport
  cfblk10 : simulink/Math Operations/MinMax Running Resettable  Function=min  vinit=0.0
  cfblk11 : Product  Inputs=*
  cfblk12 : Constant  Value=[841831262.140453]  SampleTime=1
  cfblk18 : Delay
  cfblk19 : Delay
  cfblk3 : DiscreteTransferFcn
  cfblk4 : DiscreteTransferFcn
  cfblk5 : MinMax
  cfblk6 : Bias  Bias=[-532445687.924835]
  cfblk7 : Rounding
  cfblk8 : simulink/Math Operations/MinMax Running Resettable  Function=min  vinit=0.0
  cfblk9 : Bias  Bias=[-463217681.312515]
  cfblk2 : Outport
  cfblk13 : Outport  Port=2
  cfblk14 : Outport  Port=3
  cfblk15 : Outport  Port=4
  cfblk16 : Outport  Port=5
  cfblk17 : Outport  Port=6
  wires:
  cfblk9/1 -> cfblk7/1, cfblk11/1
  cfblk8/1 -> cfblk5/1
  cfblk12/1 -> cfblk14/1
  cfblk4/1 -> cfblk15/1, cfblk6/1
  cfblk5/1 -> cfblk16/1, cfblk10/2
  cfblk3/1 -> cfblk4/1
  cfblk11/1 -> cfblk13/1, cfblk2/1, cfblk19/1
  cfblk7/1 -> cfblk17/1, cfblk8/2
  cfblk1/1 -> cfblk8/1
  cfblk10/1 -> cfblk3/1
  cfblk6/1 -> cfblk18/1
  cfblk18/1 -> cfblk10/1
  cfblk19/1 -> cfblk9/1

== system Sample594/cfblk11/cfblk19/cfblk7/cfblk8 ==
  cfblk1 : Inport
  cfblk9 : Inport  Port=2
  cfblk3 : DiscreteTransferFcn
  cfblk4 : simulink/Discrete/Difference  ICPrevInput=0.0  OutMin=[]  OutMax=[]  OutDataTypeStr=Inherit: Inherit via back propagation  OutDataType=fixdt(1, 16)  OutScaling=2^-10  DoSatur=off
  cfblk5 : simulink/Discrete/Transfer Fcn First Order  PoleZ=0.95  ICPrevOutput=0.0  DoSatur=off
  cfblk6 : Product  Inputs=**
  cfblk7 : Sin  TimeSource=Use external signal  SampleTime=0
  cfblk8 : Constant  Value=[716213657.813498]  SampleTime=1
  cfblk2 : Outport
  cfblk10 : Outport  Port=2
  wires:
  cfblk3/1 -> cfblk6/1
  cfblk9/1 -> cfblk7/1
  cfblk7/1 -> cfblk4/1
  cfblk6/1 -> cfblk2/1
  cfblk8/1 -> cfblk6/2
  cfblk4/1 -> cfblk5/1
  cfblk5/1 -> cfblk10/1
  cfblk1/1 -> cfblk3/1

== system Sample594/cfblk12/cfblk10/cfblk10/cfblk8 ==
  cfblk1 : Inport
  cfblk6 : Inport  Port=2
  cfblk7 : Inport  Port=3
  cfblk8 : Inport  Port=4
  cfblk3 : pid_lib/PID Controller  Controller=PID  Form=Parallel  TimeDomain=Discrete-time  UseExternalTs=off  SampleTime=-1  IntegratorMethod=Forward Euler  FilterMethod=Forward Euler  ControllerParametersSource=internal  P=1  I=1  D=0  UseFilter=on  N=100  TunerSelectOption=Transfer Function Based (PID Tuner App)  InitialConditionSource=internal  InitialConditionForIntegrator=0  InitialConditionForFilter=0  DifferentiatorICPrevScaledInput=0  ExternalReset=none  TrackingMode=off  Kt=1  LimitOutput=off  SatLimitsSource=internal  UpperSaturationLimit=inf  LowerSaturationLimit=-inf  LinearizeAsGain=off  AntiWindupMode=none  Kb=1  POutMin=[]  POutMax=[]  IOutMin=[]  IOutMax=[]  DOutMin=[]  DOutMax=[]  NOutMin=[]  NOutMax=[]  SumOutMin=[]  SumOutMax=[]  SaturationOutMin=[]  SaturationOutMax=[]  PParamMin=[]  PParamMax=[]  IParamMin=[]  IParamMax=[]  DParamMin=[]  DParamMax=[]  NParamMin=[]  NParamMax=[]  KbParamMin=[]  KbParamMax=[]  KtParamMin=[]  KtParamMax=[]  KbOutMin=[]  KbOutMax=[]  KtOutMin=[]  KtOutMax=[]  IntegratorOutMin=[]  IntegratorOutMax=[]  FilterOutMin=[]  FilterOutMax=[]  SumI1OutMin=[]  SumI1OutMax=[]  SumI2OutMin=[]  SumI2OutMax=[]  SumI3OutMin=[]  SumI3OutMax=[]  SumI4OutMin=[]  SumI4OutMax=[]  SumDOutMin=[]  SumDOutMax=[]  DifferentiatorOutMin=[]  DifferentiatorOutMax=[]  FilterDiffOutCoefMin=[]  FilterDiffOutCoefMax=[]  ReciprocalOutMin=[]  ReciprocalOutMax=[]  SumDenOutMin=[]  SumDenOutMax=[]  SumNumOutMin=[]  SumNumOutMax=[]  DivideOutMin=[]  DivideOutMax=[]  UdiffTsProdOutMin=[]  UdiffTsProdOutMax=[]  NTsProdOutMin=[]  NTsProdOutMax=[]  UintegralTsProdOutMin=[]  UintegralTsProdOutMax=[]  UngainTsProdOutMin=[]  UngainTsProdOutMax=[]  IntegratorContinuousStateAttributes=''  IntegratorStateMustResolveToSignalObject=off  IntegratorRTWStateStorageClass=Auto  FilterContinuousStateAttributes=''  FilterStateMustResolveToSignalObject=off  FilterRTWStateStorageClass=Auto  ParallelPVariant=InternalParameters  IdealPVariant=Disabled  IVariant=InternalParameters  DVariant=InternalParameters  IntegratorVariant=Discrete  SatVariant=Disabled  AWVariant=Passthrough  PCopyVariant=Disabled  TRVariant=Disabled  FdbkBlocksVariant=Forward  IdealPFdbkVariant=Disabled  SatFdbkVariant=Disabled  DerivativeFilterVariant=ForwardEulerFilter  NVariant=InternalParameters  NCopyVariant=Disabled  FilterICVariant=InternalICsFilter  IntegratorICVariant=InternalICs  ExternalResetVariant=Disabled  TRSumVariant=Passthrough  SumFdbkVariant=Disabled  SumVariant=Sum_PID  TsampFilterVariant=InternalTs  TsampNgainVariant=Passthrough  TsampIntegralVariant=Passthrough  ExternalSaturationOutDataTypeStr=Inherit: Same as second input
  cfblk4 : Delay  DelayLengthSource=Input port
      settings: InputPortMap=u0,p1
  cfblk5 : DiscreteFir
  cfblk9 : Delay
  cfblk2 : Outport
  wires:
  cfblk3/1 -> cfblk5/1
  cfblk6/1 -> cfblk2/1
  cfblk8/1 -> cfblk4/1
  cfblk5/1 -> cfblk4/2
  cfblk4/1 -> cfblk9/1
  cfblk9/1 -> cfblk3/1

== system Sample594/cfblk12/cfblk10/cfblk10/cfblk9 ==
  cfblk1 : Inport
  cfblk10 : Delay
  cfblk3 : UnitDelay  SampleTime=-1  HasFrameUpgradeWarning=on
  cfblk4 : Sqrt  SaturateOnIntegerOverflow=on
  cfblk5 : Sum  Inputs=+-
  cfblk6 : Polyval  Coefs=[ +2.081618890e-019, -1.441693666e-014, +4.719686976e-010, -8.536869453e-006, +1.621573104e-001, -8.087801117e+001 ]
  cfblk7 : Sum  Inputs=+
  cfblk8 : Constant  Value=[562864356.531112]  SampleTime=1
  cfblk2 : Outport
  cfblk9 : Outport  Port=2
  wires:
  cfblk8/1 -> cfblk3/1, cfblk4/1
  cfblk1/1 -> cfblk9/1
  cfblk3/1 -> cfblk2/1
  cfblk7/1 -> cfblk6/1
  cfblk4/1 -> cfblk5/1
  cfblk5/1 -> cfblk7/1
  cfblk6/1 -> cfblk10/1
  cfblk10/1 -> cfblk5/2

== system Sample594/cfblk12/cfblk10/cfblk9/cfblk9 ==
  cfblk1 : Inport
  cfblk10 : DotProduct  InputSameDT=on  OutDataTypeStr=Inherit: Inherit via internal rule
  cfblk11 : Sin  TimeSource=Use external signal  SampleTime=0
  cfblk12 : Constant  Value=[665556444.177446]  SampleTime=1
  cfblk13 : Delay
  cfblk3 : DiscreteZeroPole  Poles=[0 0.5]  Gain=1  SampleTime=-1
  cfblk4 : pid_lib/PID Controller  Controller=PID  Form=Parallel  TimeDomain=Discrete-time  UseExternalTs=off  SampleTime=-1  IntegratorMethod=Forward Euler  FilterMethod=Forward Euler  ControllerParametersSource=internal  P=1  I=1  D=0  UseFilter=on  N=100  TunerSelectOption=Transfer Function Based (PID Tuner App)  InitialConditionSource=internal  InitialConditionForIntegrator=0  InitialConditionForFilter=0  DifferentiatorICPrevScaledInput=0  ExternalReset=none  TrackingMode=off  Kt=1  LimitOutput=off  SatLimitsSource=internal  UpperSaturationLimit=inf  LowerSaturationLimit=-inf  LinearizeAsGain=off  AntiWindupMode=none  Kb=1  POutMin=[]  POutMax=[]  IOutMin=[]  IOutMax=[]  DOutMin=[]  DOutMax=[]  NOutMin=[]  NOutMax=[]  SumOutMin=[]  SumOutMax=[]  SaturationOutMin=[]  SaturationOutMax=[]  PParamMin=[]  PParamMax=[]  IParamMin=[]  IParamMax=[]  DParamMin=[]  DParamMax=[]  NParamMin=[]  NParamMax=[]  KbParamMin=[]  KbParamMax=[]  KtParamMin=[]  KtParamMax=[]  KbOutMin=[]  KbOutMax=[]  KtOutMin=[]  KtOutMax=[]  IntegratorOutMin=[]  IntegratorOutMax=[]  FilterOutMin=[]  FilterOutMax=[]  SumI1OutMin=[]  SumI1OutMax=[]  SumI2OutMin=[]  SumI2OutMax=[]  SumI3OutMin=[]  SumI3OutMax=[]  SumI4OutMin=[]  SumI4OutMax=[]  SumDOutMin=[]  SumDOutMax=[]  DifferentiatorOutMin=[]  DifferentiatorOutMax=[]  FilterDiffOutCoefMin=[]  FilterDiffOutCoefMax=[]  ReciprocalOutMin=[]  ReciprocalOutMax=[]  SumDenOutMin=[]  SumDenOutMax=[]  SumNumOutMin=[]  SumNumOutMax=[]  DivideOutMin=[]  DivideOutMax=[]  UdiffTsProdOutMin=[]  UdiffTsProdOutMax=[]  NTsProdOutMin=[]  NTsProdOutMax=[]  UintegralTsProdOutMin=[]  UintegralTsProdOutMax=[]  UngainTsProdOutMin=[]  UngainTsProdOutMax=[]  IntegratorContinuousStateAttributes=''  IntegratorStateMustResolveToSignalObject=off  IntegratorRTWStateStorageClass=Auto  FilterContinuousStateAttributes=''  FilterStateMustResolveToSignalObject=off  FilterRTWStateStorageClass=Auto  ParallelPVariant=InternalParameters  IdealPVariant=Disabled  IVariant=InternalParameters  DVariant=InternalParameters  IntegratorVariant=Discrete  SatVariant=Disabled  AWVariant=Passthrough  PCopyVariant=Disabled  TRVariant=Disabled  FdbkBlocksVariant=Forward  IdealPFdbkVariant=Disabled  SatFdbkVariant=Disabled  DerivativeFilterVariant=ForwardEulerFilter  NVariant=InternalParameters  NCopyVariant=Disabled  FilterICVariant=InternalICsFilter  IntegratorICVariant=InternalICs  ExternalResetVariant=Disabled  TRSumVariant=Passthrough  SumFdbkVariant=Disabled  SumVariant=Sum_PID  TsampFilterVariant=InternalTs  TsampNgainVariant=Passthrough  TsampIntegralVariant=Passthrough  ExternalSaturationOutDataTypeStr=Inherit: Same as second input
  cfblk5 : Trigonometry
  cfblk6 : Product  Inputs=*
  cfblk7 : Sum  Inputs=+-
  cfblk8 : Rounding
  cfblk9 : Product
  cfblk2 : Outport
  wires:
  cfblk12/1 -> cfblk2/1
  cfblk4/1 -> cfblk11/1
  cfblk3/1 -> cfblk6/1
  cfblk8/1 -> cfblk5/1
  cfblk1/1 -> cfblk4/1, cfblk3/1
  cfblk6/1 -> cfblk8/1
  cfblk5/1 -> cfblk9/1
  cfblk11/1 -> cfblk10/2, cfblk7/2
  cfblk10/1 -> cfblk9/2
  cfblk9/1 -> cfblk7/1
  cfblk7/1 -> cfblk13/1
  cfblk13/1 -> cfblk10/1

== system Sample594/cfblk12/cfblk9/cfblk5/cfblk10 ==
  cfblk1 : Inport
  cfblk12 : Inport  Port=2
  cfblk13 : Inport  Port=3
  cfblk14 : Inport  Port=4
  cfblk10 : Constant  Value=[-223676042.619406]  SampleTime=1
  cfblk11 : Constant  Value=[160556374.442012]  SampleTime=1
  cfblk3 : simulink/Discrete/Difference  ICPrevInput=0.0  OutMin=[]  OutMax=[]  OutDataTypeStr=Inherit: Inherit via back propagation  OutDataType=fixdt(1, 16)  OutScaling=2^-10  DoSatur=off
  cfblk4 : UnitDelay  SampleTime=-1  HasFrameUpgradeWarning=on
  cfblk5 : Product  Inputs=**
  cfblk6 : Sum
  cfblk7 : simulink/Math Operations/Slider Gain  gain=1  low=0  high=2
  cfblk8 : Product  Inputs=*
  cfblk9 : Sqrt  Operator=rSqrt  AlgorithmType=Newton-Raphson  SaturateOnIntegerOverflow=on
  cfblk2 : Outport
  cfblk15 : Outport  Port=2
  cfblk16 : Outport  Port=3
  wires:
  cfblk14/1 -> cfblk8/1
  cfblk8/1 -> cfblk5/1
  cfblk10/1 -> cfblk9/1
  cfblk13/1 -> cfblk16/1
  cfblk7/1 -> cfblk6/1
  cfblk3/1 -> cfblk4/1
  cfblk1/1 -> cfblk7/1
  cfblk11/1 -> cfblk5/2
  cfblk5/1 -> cfblk15/1
  cfblk12/1 -> cfblk2/1
  cfblk4/1 -> cfblk6/2
  cfblk9/1 -> cfblk3/1

== system Sample594/cfblk12/cfblk9/cfblk5/cfblk11 ==
  cfblk1 : Inport
  cfblk10 : Inport  Port=2
  cfblk11 : Inport  Port=3
  cfblk12 : Inport  Port=4
  cfblk13 : Inport  Port=5
  cfblk14 : Inport  Port=6
  cfblk3 : pid_lib/PID Controller  Controller=PID  Form=Parallel  TimeDomain=Discrete-time  UseExternalTs=off  SampleTime=-1  IntegratorMethod=Forward Euler  FilterMethod=Forward Euler  ControllerParametersSource=internal  P=1  I=1  D=0  UseFilter=on  N=100  TunerSelectOption=Transfer Function Based (PID Tuner App)  InitialConditionSource=internal  InitialConditionForIntegrator=0  InitialConditionForFilter=0  DifferentiatorICPrevScaledInput=0  ExternalReset=none  TrackingMode=off  Kt=1  LimitOutput=off  SatLimitsSource=internal  UpperSaturationLimit=inf  LowerSaturationLimit=-inf  LinearizeAsGain=off  AntiWindupMode=none  Kb=1  POutMin=[]  POutMax=[]  IOutMin=[]  IOutMax=[]  DOutMin=[]  DOutMax=[]  NOutMin=[]  NOutMax=[]  SumOutMin=[]  SumOutMax=[]  SaturationOutMin=[]  SaturationOutMax=[]  PParamMin=[]  PParamMax=[]  IParamMin=[]  IParamMax=[]  DParamMin=[]  DParamMax=[]  NParamMin=[]  NParamMax=[]  KbParamMin=[]  KbParamMax=[]  KtParamMin=[]  KtParamMax=[]  KbOutMin=[]  KbOutMax=[]  KtOutMin=[]  KtOutMax=[]  IntegratorOutMin=[]  IntegratorOutMax=[]  FilterOutMin=[]  FilterOutMax=[]  SumI1OutMin=[]  SumI1OutMax=[]  SumI2OutMin=[]  SumI2OutMax=[]  SumI3OutMin=[]  SumI3OutMax=[]  SumI4OutMin=[]  SumI4OutMax=[]  SumDOutMin=[]  SumDOutMax=[]  DifferentiatorOutMin=[]  DifferentiatorOutMax=[]  FilterDiffOutCoefMin=[]  FilterDiffOutCoefMax=[]  ReciprocalOutMin=[]  ReciprocalOutMax=[]  SumDenOutMin=[]  SumDenOutMax=[]  SumNumOutMin=[]  SumNumOutMax=[]  DivideOutMin=[]  DivideOutMax=[]  UdiffTsProdOutMin=[]  UdiffTsProdOutMax=[]  NTsProdOutMin=[]  NTsProdOutMax=[]  UintegralTsProdOutMin=[]  UintegralTsProdOutMax=[]  UngainTsProdOutMin=[]  UngainTsProdOutMax=[]  IntegratorContinuousStateAttributes=''  IntegratorStateMustResolveToSignalObject=off  IntegratorRTWStateStorageClass=Auto  FilterContinuousStateAttributes=''  FilterStateMustResolveToSignalObject=off  FilterRTWStateStorageClass=Auto  ParallelPVariant=InternalParameters  IdealPVariant=Disabled  IVariant=InternalParameters  DVariant=InternalParameters  IntegratorVariant=Discrete  SatVariant=Disabled  AWVariant=Passthrough  PCopyVariant=Disabled  TRVariant=Disabled  FdbkBlocksVariant=Forward  IdealPFdbkVariant=Disabled  SatFdbkVariant=Disabled  DerivativeFilterVariant=ForwardEulerFilter  NVariant=InternalParameters  NCopyVariant=Disabled  FilterICVariant=InternalICsFilter  IntegratorICVariant=InternalICs  ExternalResetVariant=Disabled  TRSumVariant=Passthrough  SumFdbkVariant=Disabled  SumVariant=Sum_PID  TsampFilterVariant=InternalTs  TsampNgainVariant=Passthrough  TsampIntegralVariant=Passthrough  ExternalSaturationOutDataTypeStr=Inherit: Same as second input
  cfblk4 : DiscreteTransferFcn
  cfblk5 : pid_lib/PID Controller  Controller=PID  Form=Parallel  TimeDomain=Discrete-time  UseExternalTs=off  SampleTime=-1  IntegratorMethod=Forward Euler  FilterMethod=Forward Euler  ControllerParametersSource=internal  P=1  I=1  D=0  UseFilter=on  N=100  TunerSelectOption=Transfer Function Based (PID Tuner App)  InitialConditionSource=internal  InitialConditionForIntegrator=0  InitialConditionForFilter=0  DifferentiatorICPrevScaledInput=0  ExternalReset=none  TrackingMode=off  Kt=1  LimitOutput=off  SatLimitsSource=internal  UpperSaturationLimit=inf  LowerSaturationLimit=-inf  LinearizeAsGain=off  AntiWindupMode=none  Kb=1  POutMin=[]  POutMax=[]  IOutMin=[]  IOutMax=[]  DOutMin=[]  DOutMax=[]  NOutMin=[]  NOutMax=[]  SumOutMin=[]  SumOutMax=[]  SaturationOutMin=[]  SaturationOutMax=[]  PParamMin=[]  PParamMax=[]  IParamMin=[]  IParamMax=[]  DParamMin=[]  DParamMax=[]  NParamMin=[]  NParamMax=[]  KbParamMin=[]  KbParamMax=[]  KtParamMin=[]  KtParamMax=[]  KbOutMin=[]  KbOutMax=[]  KtOutMin=[]  KtOutMax=[]  IntegratorOutMin=[]  IntegratorOutMax=[]  FilterOutMin=[]  FilterOutMax=[]  SumI1OutMin=[]  SumI1OutMax=[]  SumI2OutMin=[]  SumI2OutMax=[]  SumI3OutMin=[]  SumI3OutMax=[]  SumI4OutMin=[]  SumI4OutMax=[]  SumDOutMin=[]  SumDOutMax=[]  DifferentiatorOutMin=[]  DifferentiatorOutMax=[]  FilterDiffOutCoefMin=[]  FilterDiffOutCoefMax=[]  ReciprocalOutMin=[]  ReciprocalOutMax=[]  SumDenOutMin=[]  SumDenOutMax=[]  SumNumOutMin=[]  SumNumOutMax=[]  DivideOutMin=[]  DivideOutMax=[]  UdiffTsProdOutMin=[]  UdiffTsProdOutMax=[]  NTsProdOutMin=[]  NTsProdOutMax=[]  UintegralTsProdOutMin=[]  UintegralTsProdOutMax=[]  UngainTsProdOutMin=[]  UngainTsProdOutMax=[]  IntegratorContinuousStateAttributes=''  IntegratorStateMustResolveToSignalObject=off  IntegratorRTWStateStorageClass=Auto  FilterContinuousStateAttributes=''  FilterStateMustResolveToSignalObject=off  FilterRTWStateStorageClass=Auto  ParallelPVariant=InternalParameters  IdealPVariant=Disabled  IVariant=InternalParameters  DVariant=InternalParameters  IntegratorVariant=Discrete  SatVariant=Disabled  AWVariant=Passthrough  PCopyVariant=Disabled  TRVariant=Disabled  FdbkBlocksVariant=Forward  IdealPFdbkVariant=Disabled  SatFdbkVariant=Disabled  DerivativeFilterVariant=ForwardEulerFilter  NVariant=InternalParameters  NCopyVariant=Disabled  FilterICVariant=InternalICsFilter  IntegratorICVariant=InternalICs  ExternalResetVariant=Disabled  TRSumVariant=Passthrough  SumFdbkVariant=Disabled  SumVariant=Sum_PID  TsampFilterVariant=InternalTs  TsampNgainVariant=Passthrough  TsampIntegralVariant=Passthrough  ExternalSaturationOutDataTypeStr=Inherit: Same as second input
  cfblk6 : Sum
  cfblk7 : Sin  TimeSource=Use external signal  SampleTime=0
  cfblk8 : Constant  Value=[134067273.442335]  SampleTime=1
  cfblk9 : Constant  Value=[864688629.207743]  SampleTime=1
  cfblk2 : Outport
  cfblk15 : Outport  Port=2
  cfblk16 : Outport  Port=3
  wires:
  cfblk12/1 -> cfblk2/1
  cfblk13/1 -> cfblk15/1
  cfblk10/1 -> cfblk5/1
  cfblk3/1 -> cfblk6/1
  cfblk8/1 -> cfblk7/1
  cfblk9/1 -> cfblk3/1
  cfblk14/1 -> cfblk4/1
  cfblk6/1 -> cfblk16/1
  cfblk4/1 -> cfblk6/2

== system Sample594/cfblk12/cfblk9/cfblk5/cfblk15 ==
  cfblk1 : Inport
  cfblk11 : Inport  Port=2
  Action Port : ActionPort  ActionPortLabel=if(u1 >= 0)
  cfblk10 : Constant  Value=[35248324.032237]  SampleTime=1
  cfblk13 : Delay
  cfblk3 : DiscreteTransferFcn
  cfblk4 : Reshape
  cfblk5 : Trigonometry
  cfblk6 : Rounding
  cfblk7 : DotProduct  InputSameDT=on  OutDataTypeStr=Inherit: Inherit via internal rule
  cfblk8 : Constant  Value=[-985405299.640863]  SampleTime=1
  cfblk9 : Constant  Value=[613266480.582196]  SampleTime=1
  cfblk2 : Outport
  cfblk12 : Outport  Port=2
  wires:
  cfblk7/1 -> cfblk4/1
  cfblk10/1 -> cfblk6/1
  cfblk11/1 -> cfblk2/1
  cfblk6/1 -> cfblk5/1
  cfblk1/1 -> cfblk3/1
  cfblk9/1 -> cfblk12/1
  cfblk3/1 -> cfblk7/1
  cfblk4/1 -> cfblk13/1
  cfblk13/1 -> cfblk7/2

== system Sample594/cfblk12/cfblk9/cfblk5/cfblk16 ==
  cfblk1 : Inport
  cfblk14 : Inport  Port=2
  cfblk15 : Inport  Port=3
  Action Port : ActionPort  ActionPortLabel=else
  cfblk10 : Math  Operator=hermitian  SaturateOnIntegerOverflow=on
  cfblk11 : Polyval  Coefs=[ +2.081618890e-019, -1.441693666e-014, +4.719686976e-010, -8.536869453e-006, +1.621573104e-001, -8.087801117e+001 ]
  cfblk12 : Signum
  cfblk13 : Constant  Value=[-411477328.378402]  SampleTime=1
  cfblk17 : Delay
  cfblk3 : DiscreteZeroPole  Poles=[0 0.5]  Gain=1  SampleTime=-1
  cfblk4 : DiscreteFilter
  cfblk5 : simulink/Discrete/Transfer Fcn First Order  PoleZ=0.95  ICPrevOutput=0.0  DoSatur=off
  cfblk6 : MinMax  Function=max  Inputs=2
  cfblk7 : UnaryMinus
  cfblk8 : Assignment  DiagnosticForDimensions=Warning  IndexOptions=Index vector (dialog)  Indices=1  OutputSizes=1
  cfblk9 : Reshape
  cfblk2 : Outport
  cfblk16 : Outport  Port=2
  wires:
  cfblk11/1 -> cfblk7/1
  cfblk9/1 -> cfblk12/1
  cfblk14/1 -> cfblk5/1
  cfblk4/1 -> cfblk3/1
  cfblk10/1 -> cfblk11/1
  cfblk3/1 -> cfblk8/1
  cfblk13/1 -> cfblk2/1
  cfblk1/1 -> cfblk4/1
  cfblk8/1 -> cfblk6/1
  cfblk15/1 -> cfblk16/1
  cfblk7/1 -> cfblk9/1
  cfblk5/1 -> cfblk6/2
  cfblk6/1 -> cfblk10/1
  cfblk12/1 -> cfblk17/1
  cfblk17/1 -> cfblk8/2
